simulink model "RC_control"  (Simulink 6.6)
settings: Solver=FixedStepDiscrete  StartTime=0.0  StopTime=10.0  FixedStep=0.001  RelTol=1e-3
undefined symbols (not defined in the file): DiscIntNeverNeededParam, ecan1_init, ecan1_transmit_matlab, OC2max, u1
libraries: simulink x26, dsPICdrivers x11
(part 1 of 2)
settings Model: Creator=Administrator  LastModifiedBy=bwmairs  ProdHWDeviceType=16-bit Generic
settings OptimizationCC: OptimizeModelRefInitCode=on  LifeSpan=1
settings HardwareCC: ProdBitPerInt=16  ProdEndianess=LittleEndian  ProdWordSize=16  ProdHWDeviceType=16-bit Generic  TargetHWDeviceType=32-bit Generic
settings RTWCC: SystemTargetFile=dspic.tlc  TemplateMakefile=dspic_pic30_gcc.tmf  PostCodeGenCommand=dsPIC_Compile()  Description=Embedded Target for Microchip dsPIC (real-time)  ProcessScript=dspic_make_rtw_hook
settings RTWCC: CustomSource=|
  | ../../../../ecan/circBuffer.c
  | ../../../../ecan/ecanFunctions.c
settings RTWCC: CustomInitializer=|
  | #include "InCap.h"
  | #include <p33fxxxx.h>
  |     T5CONbits.TON = 0; // Stop any 16-bit Timer5 operation
  |     T4CONbits.TON = 0; // Stop any 16/32-bit Timer4 operation
  |     T4CONbits.T32 = 1; // Enable 32-bit Timer mode
  |     T4CONbits.TCS = 0; // Select internal instruction cycle clock
  |     T4CONbits.TGATE = 0; // Disable Gated Timer mode
  |     T4CONbits.TCKPS = 0b00;// Select 1:1 Prescaler
  |     TMR5 = 0x00; // Clear 32-bit Timer (msw)
  |     TMR4 = 0x00; // Clear 32-bit Timer (lsw)
  |     PR5 = 0x0010; // Load 32-bit period value (msw)
  |     PR4 = 0x0000; // Load 32-bit period value (lsw)
  |     IPC7bits.T5IP = 0x01; // Set Timer5 Interrupt Priority Level
  |     IFS1bits.T5IF = 0; // Clear Timer5 Interrupt Flag
  |     IEC1bits.T5IE = 1; // Enable Timer5 interrupt
  |     T4CONbits.TON = 1; // Start 32-bit Timer
  | 
  |     // Configure our input captures
  |     OpenCapture1(IC_IDLE_CON & IC_TIMER2_SRC & IC_INT_1CAPTURE &
  |                  IC_EVERY_RISE_EDGE);
  |     ConfigIntCapture1(IC_INT_ON & IC_INT_PRIOR_7);
  |     OpenCapture2(IC_IDLE_CON & IC_TIMER2_SRC & IC_INT_1CAPTURE &
  |                  IC_EVERY_RISE_EDGE);
  |     ConfigIntCapture2(IC_INT_ON & IC_INT_PRIOR_7);
  | 
  | // Configure ports D1, D5, G9 to be open-drain, as 5V outputs are needed
  | ODCGbits.ODCG9 = 1;
  | ODCDbits.ODCD5 = 1;
  | ODCDbits.ODCD1 = 1;
  | 
  | // Enable serial output
  | U2STAbits.UTXEN = 1;
settings CodeAppCC: IgnoreCustomStorageClasses=off
settings STFCustomTargetCC: TargetFcnLib=ansi_tfl_tmw.mat  GenFloatMathFcnCalls=ANSI_C  ModelReferenceCompliant=off  IncludeMdlTerminateFcn=off  CombineOutputUpdateFcns=on  SuppressErrorStatus=on  ERTCustomFileBanners=on  SupportContinuousTime=off  SupportNonInlinedSFcns=off  SystemTargetFile=dspic.tlc
settings ERTTargetCC: TargetFcnLib=ansi_tfl_tmw.mat  GenFloatMathFcnCalls=ANSI_C  ModelReferenceCompliant=off  IncludeMdlTerminateFcn=off  SuppressErrorStatus=on  ModelStepFunctionPrototypeControlCompliant=off  ExtModeMexFile=noextcomm  InlinedParameterPlacement=NonHierarchical  ERTSrcFileBannerTemplate=dsPIC_code_template.cgt  ERTHdrFileBannerTemplate=dsPIC_code_template.cgt  ERTDataSrcFileTemplate=dsPIC_code_template.cgt  ERTDataHdrFileTemplate=dsPIC_code_template.cgt  ERTCustomFileTemplate=dsPIC_main.tlc
settings CustomProperty: DataType=string  Value=C:\PROGRA~1\MATLAB\R2007a\bin\win32\gmake

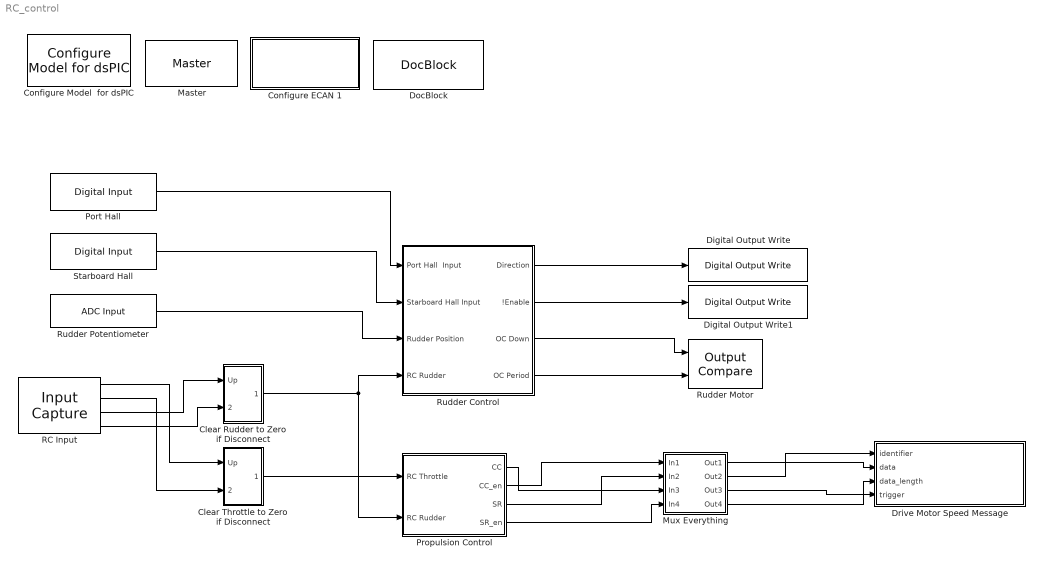
== system RC_control ==
  Clear Rudder to Zero if Disconnect : Subsystem
  Clear Throttle to Zero if Disconnect : Subsystem
  Configure ECAN 1 : Subsystem  mask(Initialize ECAN 1){frame_setting=off, mode=Normal, dma_rx_chan=2, dma_tx_chan=0, baud=250000, ps1=8, pd=5, ps2=6, sjw=4, tq=20, triple_sample=on, dma_buf_size=6 buffers, rx_bufs=[], tx_bufs=[0], buf_0_tx_pri=Highest, buf_0_rte=No, buf_1_tx_pri=Highest, buf_1_rte=No, buf_2_tx_pri=Lowest, buf_2_rte=No, buf_3_tx_pri=Lowest, buf_3_rte=No, buf_4_tx_pri=Lowest, buf_4_rte=No, buf_5_tx_pri=Lowest, buf_5_rte=No, buf_6_tx_pri=Lowest, buf_6_rte=No, buf_7_tx_pri=Lowest, buf_7_rte=No, mask_0=0, mask_0_mide=Match std or ext, mask_1=0, mask_1_mide=Match std or ext, mask_2=0, mask_2_mide=Match std or ext, filters=[], filter_0=hex2dec('400'), filter_0_mask=0, filter_0_exide=Match only standard, filter_0_buf=1, filter_1=hex2dec('401'), filter_1_mask=0, filter_1_exide=Match only standard, filter_1_buf=2, filter_2=hex2dec('402'), filter_2_mask=0, filter_2_exide=Match only standard, filter_2_buf=3, filter_3=0, filter_3_mask=0, filter_3_exide=Match only standard, filter_3_buf=0, filter_4=0, filter_4_mask=0, filter_4_exide=Match only standard, filter_4_buf=0, filter_5=0, filter_5_mask=0, filter_5_exide=Match only standard, filter_5_buf=0, filter_6=0, filter_6_mask=0, filter_6_exide=Match only standard, filter_6_buf=0, filter_7=0, filter_7_mask=0, filter_7_exide=Match only standard, filter_7_buf=0, filter_8=0, filter_8_mask=0, filter_8_exide=Match only standard, filter_8_buf=0, filter_9=0, filter_9_mask=<empty>, filter_9_exide=Match only standard, filter_9_buf=0, filter_10=0, filter_10_mask=0, filter_10_exide=Match only standard, filter_10_buf=0, filter_11=0, filter_11_mask=0, filter_11_exide=Match only standard, filter_11_buf=0, filter_12=0, filter_12_mask=0, filter_12_exide=Match only standard, filter_12_buf=0, filter_13=0, filter_13_mask=0, filter_13_exide=Match only standard, filter_13_buf=0, filter_14=0, filter_14_mask=0, filter_14_exide=Match only standard, filter_14_buf=0, filter_15=0, filter_15_mask=0, filter_15_exide=Match only standard, filter_15_buf=0}
      mask prompts: frame_setting "Extended Frames (Standard if unchecked)"; dma_rx_chan "DMA Reception Channel"; dma_tx_chan "DMA Transmission Channel"; baud "Baud Rate (bps)"; ps1 "Phase Segment 1"; pd "Propagation Delay"; ps2 "Phase Segment 2"; sjw "Sync Jump Width"; tq "Time Quanta"; triple_sample "Triple-sample"; dma_buf_size "DMA Buffer Size"; rx_bufs "Reception Buffers"; tx_bufs "Transmission Buffers"; buf_0_tx_pri "Buffer 0 Transmission Priority"; buf_0_rte "Buffer 0 Remote Transmit Enable"; buf_1_tx_pri "Buffer 1 Transmission Priority"; buf_1_rte "Buffer 1 Remote Transmit Enable"; buf_2_tx_pri "Buffer 2 Transmission Priority"; buf_2_rte "Buffer 2 Remote Transmit Enable"; buf_3_tx_pri "Buffer 3 Transmission Priority"; buf_3_rte "Buffer 3 Remote Transmit Enable"; buf_4_tx_pri "Buffer 4 Transmission Priority"; buf_4_rte "Buffer 4 Remote Transmit Enable"; buf_5_tx_pri "Buffer 5 Transmission Priority"; buf_5_rte "Buffer 5 Remote Transmit Enable"; buf_6_tx_pri "Buffer 6 Transmission Priority"; buf_6_rte "Buffer 6 Remote Transmit Enable"; buf_7_tx_pri "Buffer 7 Transmission Priority"; buf_7_rte "Buffer 7 Remote Transmit Enable"; mask_0 "Mask 0"; mask_0_mide "Mask 0 Receive Mode"; mask_1 "Mask 1"; mask_1_mide "Mask 1 Receive Mode"; mask_2 "Mask 2"; mask_2_mide "Mask 2 Receive Mode"; filter_0 "Filter 0"; filter_0_mask "Filter 0 Mask"; filter_0_exide "Filter 0 Mode"; filter_0_buf "Filter 0 Buffer"; filter_1 "Filter 1"; filter_1_mask "Filter 1 Mask"; filter_1_exide "Filter 1 Mode"; filter_1_buf "Filter 1 Buffer"; filter_2 "Filter 2"; filter_2_mask "Filter 2 Mask"; filter_2_exide "Filter 2 Mode"; filter_2_buf "Filter 2 Buffer"; filter_3 "Filter 3"; filter_3_mask "Filter 3 Mask"; filter_3_exide "Filter 3 Mode"; filter_3_buf "Filter 3 Buffer"; filter_4 "Filter 4"; filter_4_mask "Filter 4 Mask"; filter_4_exide "Filter 4 Mode"; filter_4_buf "Filter 4 Buffer"; filter_5 "Filter 5"; filter_5_mask "Filter 5 Mask"; filter_5_exide "Filter 5 Mode"; filter_5_buf "Filter 5 Buffer"; filter_6 "Filter 6"; filter_6_mask "Filter 6 Mask"; filter_6_exide "Filter 6 Mode"; filter_6_buf "Filter 6 Buffer"; filter_7 "Filter 7"; filter_7_mask "Filter 7 Mask"; filter_7_exide "Filter 7 Mode"; filter_7_buf "Filter 7 Buffer"; filter_8 "Filter 8"; filter_8_mask "Filter 8 Mask"; filter_8_exide "Filter 8 Mode"; filter_8_buf "Filter 8 Buffer"; filter_9 "Filter 9"; filter_9_mask "Filter 9 Mask"; filter_9_exide "Filter 9 Mode"; filter_9_buf "Filter 9 Buffer"; filter_10 "Filter 10"; filter_10_mask "Filter 10 Mask"; filter_10_exide "Filter 10 Mode"; filter_10_buf "Filter 10 Buffer"; filter_11 "Filter 11"; filter_11_mask "Filter 11 Mask"; filter_11_exide "Filter 11 Mode"; filter_11_buf "Filter 11 Buffer"; filter_12 "Filter 12"; filter_12_mask "Filter 12 Mask"; filter_12_exide "Filter 12 Mode"; filter_12_buf "Filter 12 Buffer"; filter_13 "Filter 13"; filter_13_mask "Filter 13 Mask"; filter_13_exide "Filter 13 Mode"; filter_13_buf "Filter 13 Buffer"; filter_14 "Filter 14"; filter_14_mask "Filter 14 Mask"; filter_14_exide "Filter 14 Mode"; filter_14_buf "Filter 14 Buffer"; filter_15 "Filter 15"; filter_15_mask "Filter 15 Mask"; filter_15_exide "Filter 15 Mode"; filter_15_buf "Filter 15 Buffer"
      mask help: Initializes the ECAN 1 module on the dsPIC33f. Allows for configuration of almost all ECAN options to produce a usable system.
      mask init:
      | parameters = uint16(zeros(53,1));
      | 
      | %% Generate parameter 1
      | parameters(1) = frame_setting;
      | mode_id = 0;
      | switch mode
      |     case 'Disabled'
      |         mode_id = 1;
      |     case 'Loopback'
      |         mode_id = 2;
      |     case 'Listen only'
      |         mode_id = 3;
      |     case 'Listen all'
      |         mode_id = 7;
      | end
      | parameters(1) = bitor(parameters(1), bitshift(mode_id, 2));
      | parameters(1) = bitor(parameters(1), bitshift(dma_rx_chan, 5));
      | parameters(1) = bitor(parameters(1), bitshift(dma_tx_chan, 8));
      | 
      | %% Generate parameter 2
      | parameters(2) = baud / 100;
      | 
      | %% Generate parameter 3
      | h = find_system(bdroot(gcb),'FollowLinks','on','LookUnderMasks','all','Tag','dsPIC_MASTER');
      | fcy = 0;
      | if ~isempty(h)
      |     OverrideFcy = strcmp(get_param(h{1},'OverrideFcy'),'on');
      |     if (OverrideFcy == 1)
      |         fcy = str2num(get_param(h{1},'NewFcy'));     %% overridded fcy
      |     else
      |         fcy = str2num(get_param(h{1},'fcy'));
      |     end 
      | end
      | parameters(3) = fcy / 1000;
      | 
      | %% Generate parameter 4
      | parameters(4) = ps1 - 1;
      | parameters(4) = bitor(parameters(4), bitshift(pd - 1, 3));
      | parameters(4) = bitor(parameters(4), bitshift(ps2 - 1, 6));
      | parameters(4) = bitor(parameters(4), bitshift(sjw - 1, 9));
      | if triple_sample == 1
      |     parameters(4) = bitset(parameters(4),12);
      | end
      | 
      | %% Generate parameter 5
      | for k = 1:length(filters)
      |     parameters(5) = bitset(parameters(5),filters(k)+1);
      | end;
      | 
      | % Map filter mask values into proper values
      | filter_masks = [filter_0_mask; filter_1_mask; filter_2_mask; filter_3_mask; filter_4_mask; filter_5_mask; filter_6_mask; filter_7_mask; filter_8_mask; filter_9_mask; filter_10_mask; filter_11_mask; filter_12_mask; filter_13_mask; filter_14_mask; filter_15_mask;];
      | filter_masks = filter_masks - 2;
      | filter_masks(filter_masks == -1) = 3;
      | 
      | %% Generate parameters 6 and 7
      | for k = 1:length(filters);
      |     filter = filters(k) + 1;
      |     if filter < 9
      |         parameters(6) = bitor(parameters(6), bitshift(filter_masks(filter),2*(filter-1)));
      |     else
      |         parameters(7) = bitor(parameters(7), bitshift(filter_masks(filter),2*(filter-9)));
      |     end
      | end
      | 
      | % Generate parameters 8 and 9
      | parameters(8) = bitshift(bitand(mask_0,hex2dec('18000000')),-27); % EID17-16
      | parameters(8) = bitor(parameters(8), bitshift(bitand(mask_0,hex2dec('7FF')), 5)); % SID
      | parameters(8) = bitor(parameters(8), bitshift(mask_0_mide - 1, 3)); % MIDE
      | parameters(9) = bitshift(bitand(mask_0,hex2dec('7FFF800')),-11); % EID15-0
      | 
      | %% Generate parameters 10 and 11
      | parameters(10) = bitshift(bitand(mask_1,hex2dec('18000000')),-27); % EID17-16
      | parameters(10) = bitor(parameters(10), bitshift(bitand(mask_1,hex2dec('7FF')), 5)); % SID
      | parameters(10) = bitor(parameters(10), bitshift(mask_1_mide - 1, 3)); % MIDE
      | parameters(11) = bitshift(bitand(mask_1,hex2dec('7FFF800')),-11); % EID15-0
      | 
      | %% Generate parameters 12 and 13
      | parameters(12) = bitshift(bitand(mask_2,hex2dec('18000000')),-27); % EID17-16
      | parameters(12) = bitor(parameters(12), bitshift(bitand(mask_2,hex2dec('7FF')), 5)); % SID
      | parameters(12) = bitor(parameters(12), bitshift(mask_2_mide - 1, 3)); % MIDE
      | parameters(13) = bitshift(bitand(mask_2,hex2dec('7FFF800')),-11); % EID15-0
      | 
      | % Generate parameters 14-17
      | buf_priorities = [buf_0_tx_pri;buf_1_tx_pri;buf_2_tx_pri;buf_3_tx_pri;buf_4_tx_pri;buf_5_tx_pri;buf_6_tx_pri;buf_7_tx_pri] - 1;
      | buf_rtes = [buf_0_rte;buf_1_rte;buf_2_rte;buf_3_rte;buf_4_rte;buf_5_rte;buf_6_rte;buf_7_rte] - 1;
      | 
      | % Create a vector of chars to modify
      | regs = uint16(zeros(8,1));
      | 
      | % Go through all enabled transmission buffers setting appropriate bits
      | for b = 1:size(tx_bufs,1)
      |     
      |     index = tx_bufs(b) + 1;
      |     
      |     % Set transmission bit
      |     regs(index) = bitset(regs(index),8);
      | 
      |     % Set priority bits
      |     regs(index) = bitor(regs(index), buf_priorities(index));
      | 
      |     % Set remote transmit enable bits
      |     if buf_rtes(index) == 1
      |         regs(index) = bitset(regs(index),3);
      |     end
      | end
      | 
      | for b = 1:size(rx_bufs,1)
      |     
      |     index = rx_bufs(b) + 1;
      | 
      |     % Set priority bits
      |     regs(index) = bitor(regs(index), buf_priorities(index));
      | 
      |     % Set remote transmit enable bits
      |     if buf_rtes(index) == 1
      |         regs(index) = bitset(regs(index),3);
      |     end
      | end
      | 
      | % Map our matrix into registers
      | parameters(14) = bitor(bitshift(regs(2),8), regs(1));
      | parameters(15) = bitor(bitshift(regs(4),8), regs(3));
      | parameters(16) = bitor(bitshift(regs(6),8), regs(5));
      | parameters(17) = bitor(bitshift(regs(8),8), regs(7));
      | 
      | % Map the filter buffer values to corresponding bit values
      | filter_buffers = [filter_0_buf; filter_1_buf; filter_2_buf; filter_3_buf; filter_4_buf; filter_5_buf; filter_6_buf; filter_7_buf; filter_8_buf; filter_9_buf; filter_10_buf; filter_11_buf; filter_12_buf; filter_13_buf; filter_14_buf; filter_15_buf;];
      | filter_buffers = filter_buffers - 1;
      | 
      | %% Generate parameter 18
      | if bitget(parameters(5),1) == 1
      |     parameters(18) = filter_buffers(1);
      | end
      | if bitget(parameters(5),2) == 1
      |     parameters(18) = bitor(parameters(18), bitshift(filter_buffers(2), 4));
      | end
      | if bitget(parameters(5),3) == 1
      |     parameters(18) = bitor(parameters(18), bitshift(filter_buffers(3), 8));
      | end
      | if bitget(parameters(5),4) == 1
      |     parameters(18) = bitor(parameters(18), bitshift(filter_buffers(4), 12));
      | end
      | 
      | %% Generate parameter 19
      | if bitget(parameters(5),5) == 1
      |     parameters(19) = filter_buffers(5);
      | end
      | if bitget(parameters(5),6) == 1
      |     parameters(19) = bitor(parameters(19), bitshift(filter_buffers(6), 4));
      | end
      | if bitget(parameters(5),7) == 1
      |     parameters(19) = bitor(parameters(19), bitshift(filter_buffers(7), 8));
      | end
      | if bitget(parameters(5),8) == 1
      |     parameters(19) = bitor(parameters(19), bitshift(filter_buffers(8), 12));
      | end
      | 
      | %% Generate parameter 20
      | if bitget(parameters(5),9) == 1
      |     parameters(20) = filter_buffers(9);
      | end
      | if bitget(parameters(5),10) == 1
      |     parameters(20) = bitor(parameters(20), bitshift(filter_buffers(10), 4));
      | end
      | if bitget(parameters(5),11) == 1
      |     parameters(20) = bitor(parameters(20), bitshift(filter_buffers(11), 8));
      | end
      | if bitget(parameters(5),12) == 1
      |     parameters(20) = bitor(parameters(20), bitshift(filter_buffers(12), 12));
      | end
      | 
      | %% Generate parameter 21
      | if bitget(parameters(5),13) == 1
      |     parameters(21) = filter_buffers(13);
      | end
      | if bitget(parameters(5),14) == 1
      |     parameters(21) = bitor(parameters(21), bitshift(filter_buffers(14), 4));
      | end
      | if bitget(parameters(5),15) == 1
      |     parameters(21) = bitor(parameters(21), bitshift(filter_buffers(15), 8));
      | end
      | if bitget(parameters(5),16) == 1
      |     parameters(21) = bitor(parameters(21), bitshift(filter_buffers(16), 12));
      | end
      | 
      | % Generate parameters 22 and 23
      | parameters(22) = bitshift(bitand(filter_0,hex2dec('18000000')),-27); % EID17-16
      | parameters(22) = bitor(parameters(22), bitshift(bitand(filter_0,hex2dec('7FF')), 5)); % SID
      | parameters(22) = bitor(parameters(22), bitshift(filter_0_exide - 1, 3)); % EXIDE
      | parameters(23) = bitshift(bitand(uint32(filter_0),hex2dec('7FFF800')),-11); % EID15-0
      | 
      | %% Generate parameters 24 and 25
      | parameters(24) = bitshift(bitand(filter_1,hex2dec('18000000')),-27); % EID17-16
      | parameters(24) = bitor(parameters(24), bitshift(bitand(filter_1,hex2dec('7FF')), 5)); % SID
      | parameters(24) = bitor(parameters(24), bitshift(filter_1_exide - 1, 3)); % EXIDE
      | parameters(25) = bitshift(bitand(uint32(filter_1),hex2dec('7FFF800')),-11); % EID15-0
      | 
      | %% Generate parameters 26 and 27
      | parameters(26) = bitshift(bitand(filter_2,hex2dec('18000000')),-27); % EID17-16
      | parameters(26) = bitor(parameters(26), bitshift(bitand(filter_2,hex2dec('7FF')), 5)); % SID
      | parameters(26) = bitor(parameters(26), bitshift(filter_2_exide - 1, 3)); % EXIDE
      | parameters(27) = bitshift(bitand(uint32(filter_2),hex2dec('7FFF800')),-11); % EID15-0
      | 
      | %% Generate parameters 28 and 29
      | parameters(28) = bitshift(bitand(filter_3,hex2dec('18000000')),-27); % EID17-16
      | parameters(28) = bitor(parameters(28), bitshift(bitand(filter_3,hex2dec('7FF')), 5)); % SID
      | parameters(28) = bitor(parameters(28), bitshift(filter_3_exide - 1, 3)); % EXIDE
      | parameters(29) = bitshift(bitand(uint32(filter_3),hex2dec('7FFF800')),-11); % EID15-0
      | 
      | %% Generate parameters 30 and 31
      | parameters(30) = bitshift(bitand(filter_4,hex2dec('18000000')),-27); % EID17-16
      | parameters(30) = bitor(parameters(30), bitshift(bitand(filter_4,hex2dec('7FF')), 5)); % SID
      | parameters(30) = bitor(parameters(30), bitshift(filter_4_exide - 1, 3)); % EXIDE
      | parameters(31) = bitshift(bitand(uint32(filter_4),hex2dec('7FFF800')),-11); % EID15-0
      | 
      | %% Generate parameters 32 and 33
      | parameters(32) = bitshift(bitand(filter_5,hex2dec('18000000')),-27); % EID17-16
      | parameters(32) = bitor(parameters(32), bitshift(bitand(filter_5,hex2dec('7FF')), 5)); % SID
      | parameters(32) = bitor(parameters(32), bitshift(filter_5_exide - 1, 3)); % EXIDE
      | parameters(33) = bitshift(bitand(uint32(filter_5),hex2dec('7FFF800')),-11); % EID15-0
      | 
      | %% Generate parameters 34 and 35
      | parameters(34) = bitshift(bitand(filter_6,hex2dec('18000000')),-27); % EID17-16
      | parameters(34) = bitor(parameters(34), bitshift(bitand(filter_6,hex2dec('7FF')), 5)); % SID
      | parameters(34) = bitor(parameters(34), bitshift(filter_6_exide - 1, 3)); % EXIDE
      | parameters(35) = bitshift(bitand(uint32(filter_6),hex2dec('7FFF800')),-11); % EID15-0
      | 
      | %% Generate parameters 36 and 37
      | parameters(36) = bitshift(bitand(filter_7,hex2dec('18000000')),-27); % EID17-16
      | parameters(36) = bitor(parameters(36), bitshift(bitand(filter_7,hex2dec('7FF')), 5)); % SID
      | parameters(36) = bitor(parameters(36), bitshift(filter_7_exide - 1, 3)); % EXIDE
      | parameters(37) = bitshift(bitand(uint32(filter_7),hex2dec('7FFF800')),-11); % EID15-0
      | 
      | %% Generate parameters 38 and 39
      | parameters(38) = bitshift(bitand(filter_8,hex2dec('18000000')),-27); % EID17-16
      | parameters(38) = bitor(parameters(38), bitshift(bitand(filter_8,hex2dec('7FF')), 5)); % SID
      | parameters(38) = bitor(parameters(38), bitshift(filter_8_exide - 1, 3)); % EXIDE
      | parameters(39) = bitshift(bitand(uint32(filter_8),hex2dec('7FFF800')),-11); % EID15-0
      | 
      | %% Generate parameters 40 and 41
      | parameters(40) = bitshift(bitand(filter_9,hex2dec('18000000')),-27); % EID17-16
      | parameters(40) = bitor(parameters(40), bitshift(bitand(filter_9,hex2dec('7FF')), 5)); % SID
      | parameters(40) = bitor(parameters(40), bitshift(filter_9_exide - 1, 3)); % EXIDE
      | parameters(41) = bitshift(bitand(uint32(filter_9),hex2dec('7FFF800')),-11); % EID15-0
      | 
      | %% Generate parameters 42 and 43
      | parameters(42) = bitshift(bitand(filter_10,hex2dec('18000000')),-27); % EID17-16
      | parameters(42) = bitor(parameters(42), bitshift(bitand(filter_10,hex2dec('7FF')), 5)); % SID
      | parameters(42) = bitor(parameters(42), bitshift(filter_10_exide - 1, 3)); % EXIDE
      | parameters(43) = bitshift(bitand(uint32(filter_10),hex2dec('7FFF800')),-11); % EID15-0
      | 
      | %% Generate parameters 44 and 45
      | parameters(44) = bitshift(bitand(filter_11,hex2dec('18000000')),-27); % EID17-16
      | parameters(44) = bitor(parameters(44), bitshift(bitand(filter_11,hex2dec('7FF')), 5)); % SID
      | parameters(44) = bitor(parameters(44), bitshift(filter_11_exide - 1, 3)); % EXIDE
      | parameters(45) = bitshift(bitand(uint32(filter_11),hex2dec('7FFF800')),-11); % EID15-0
      | 
      | %% Generate parameters 46 and 47
      | parameters(46) = bitshift(bitand(filter_12,hex2dec('18000000')),-27); % EID17-16
      | parameters(46) = bitor(parameters(46), bitshift(bitand(filter_12,hex2dec('7FF')), 5)); % SID
      | parameters(46) = bitor(parameters(46), bitshift(filter_12_exide - 1, 3)); % EXIDE
      | parameters(47) = bitshift(bitand(uint32(filter_12),hex2dec('7FFF800')),-11); % EID15-0
      | 
      | %% Generate parameters 48 and 49
      | parameters(48) = bitshift(bitand(filter_13,hex2dec('18000000')),-27); % EID17-16
      | parameters(48) = bitor(parameters(48), bitshift(bitand(filter_13,hex2dec('7FF')), 5)); % SID
      | parameters(48) = bitor(parameters(48), bitshift(filter_13_exide - 1, 3)); % EXIDE
      | parameters(49) = bitshift(bitand(uint32(filter_13),hex2dec('7FFF800')),-11); % EID15-0
      | 
      | %% Generate parameters 50 and 51
      | parameters(50) = bitshift(bitand(filter_14,hex2dec('18000000')),-27); % EID17-16
      | parameters(50) = bitor(parameters(50), bitshift(bitand(filter_14,hex2dec('7FF')), 5)); % SID
      | parameters(50) = bitor(parameters(50), bitshift(filter_14_exide - 1, 3)); % EXIDE
      | parameters(51) = bitshift(bitand(uint32(filter_14),hex2dec('7FFF800')),-11); % EID15-0
      | 
      | %% Generate parameters 52 and 53
      | parameters(52) = bitshift(bitand(filter_15,hex2dec('18000000')),-27); % EID17-16
      | parameters(52) = bitor(parameters(52), bitshift(bitand(filter_15,hex2dec('7FF')), 5)); % SID
      | parameters(52) = bitor(parameters(52), bitshift(filter_15_exide - 1, 3)); % EXIDE
      | parameters(53) = bitshift(bitand(uint32(filter_15),hex2dec('7FFF800')),-11); % EID15-0
      mask StyleString: checkbox,popup(Disabled|Listen all|Listen only|Loopback|Normal),edit,edit,edit,edit,edit,edit,popup(1|2|3|4),edit,checkbox,popup(4 buffers|6 buffers|8 buffers|12 buffers|16 buffers|24 buffers|32 buffers),edit,edit,popup(Lowest|Low|High|Highest),popup(No|Yes),popup(Lowest|Low|High|Highest),popup(No|Yes),popup(Lowest|Low|High|Highest),popup(No|Yes),popup(Lowest|Low|High|Highest),popup(No|Yes),popup(Lowest|Low|High|Highest),popup(No|Yes),popup(Lowest|Low|High|Highest),popup(No|Yes),popup(Lowest|Low|High|Highest),popup(No|Yes),popup(Lowest|Low|High|Highest),popup(No|Yes),edit,popup(Match std or ext|Obey filter mode),edit,popup(Match std or ext|Obey filter mode),edit,popup(Match std or ext|Obey filter mode),edit,edit,popup(--|0|1|2),popup(Match only standard|Match only extended),popup(0|1|2|3|4|5|6|7|8|9|10|11|12|13|14|FIFO),edit,popup(--|0|1|2),popup(Match only standard|Match only extended),popup(0|1|2|3|4|5|6|7|8|9|10|11|12|13|14|FIFO),edit,popup(--|0|1|2),popup(Match only standard|Match only extended),popup(0|1|2|3|4|5|6|7|8|9|10|11|12|13|14|FIFO),edit,popup(--|0|1|2),popup(Match only standard|Match only extended),popup(0|1|2|3|4|5|6|7|8|9|10|11|12|13|14|FIFO),edit,popup(--|0|1|2),popup(Match only standard|Match only extended),popup(0|1|2|3|4|5|6|7|8|9|10|11|12|13|14|FIFO),edit,popup(--|0|1|2),popup(Match only standard|Match only extended),popup(0|1|2|3|4|5|6|7|8|9|10|11|12|13|14|FIFO),edit,popup(--|0|1|2),popup(Match only standard|Match only extended),popup(0|1|2|3|4|5|6|7|8|9|10|11|12|13|14|FIFO),edit,popup(--|0|1|2),popup(Match only standard|Match only extended),popup(0|1|2|3|4|5|6|7|8|9|10|11|12|13|14|FIFO),edit,popup(--|0|1|2),popup(Match only standard|Match only extended),popup(0|1|2|3|4|5|6|7|8|9|10|11|12|13|14|FIFO),edit,popup(<empty>),popup(Match only standard|Match only extended),popup(0|1|2|3|4|5|6|7|8|9|10|11|12|13|14|FIFO),edit,popup(--|0|1|2),popup(Match only standard|Match only extended),popup(0|1|2|3|4|5|6|7|8|9|10|11|12|13|14|FIFO),edit,popup(--|0|1|2),popup(Match only standard|Match only extended),popup(0|1|2|3|4|5|6|7|8|9|10|11|12|13|14|FIFO),edit,popup(--|0|1|2),popup(Match only standard|Match only extended),popup(0|1|2|3|4|5|6|7|8|9|10|11|12|13|14|FIFO),edit,popup(--|0|1|2),popup(Match only standard|Match only extended),popup(0|1|2|3|4|5|6|7|8|9|10|11|12|13|14|FIFO),edit,popup(--|0|1|2),popup(Match only standard|Match only extended),popup(0|1|2|3|4|5|6|7|8|9|10|11|12|13|14|FIFO),edit,popup(--|0|1|2),popup(Match only standard|Match only extended),popup(0|1|2|3|4|5|6|7|8|9|10|11|12|13|14|FIFO)
      mask CallbackString:
      | |||||tq = 1 + str2num(get_param(gcb, 'ps1')) + str2num(get_param(gcb, 'pd')) + str2num(get_param(gcb, 'ps2'));
      | set_param(gcb, 'tq', int2str(tq));|tq = 1 + str2num(get_param(gcb, 'ps1')) + str2num(get_param(gcb, 'pd')) + str2num(get_param(gcb, 'ps2'));
      | set_param(gcb, 'tq', int2str(tq));|tq = 1 + str2num(get_param(gcb, 'ps1')) + str2num(get_param(gcb, 'pd')) + str2num(get_param(gcb, 'ps2'));
      | set_param(gcb, 'tq', int2str(tq));||||||filters = eval(get_param(gcb,'tx_bufs'));
      | mVisibilities = get_param(gcb,'MaskVisibilities');
      | mNames = get_param(gcb,'MaskNames');
      | for i = 1:size(mNames);
      | 	n = mNames{i};
      |     if size(n,2) > 4 && strcmp(n(1:4), 'buf_') == 1
      |         filterNumber = sscanf(n, 'buf_%d');
      |         if isempty(find(filters == filterNumber, 1)) == 0
      |              mVisibilities{i} = 'on';
      |         else
      |              mVisibilities{i} = 'off';
      |         end
      |     end
      | end
      | set_param(gcb, 'MaskVisibilities', mVisibilities);|||||||||||||||||||||||filters = eval(get_param(gcb,'filters'));
      | mVisibilities = get_param(gcb,'MaskVisibilities');
      | mNames = get_param(gcb,'MaskNames');
      | for i = 1:size(mNames);
      | 	n = mNames{i};
      |     if size(n,2) > 7 && strcmp(n(1:7), 'filter_') == 1
      |         filterNumber = sscanf(n, 'filter_%d');
      |         if isempty(find(filters == filterNumber, 1)) == 0
      |              mVisibilities{i} = 'on';
      |         else
      |              mVisibilities{i} = 'off';
      |         end
      |     end
      | end
      | set_param(gcb, 'MaskVisibilities', mVisibilities);||||||||||||||||||||||||||||||||||||||||||||||||||||||||||||||||
      mask Display: text(0.5,0.5,'Configure ECAN1','horizontalAlignment','center','verticalAlignment','middle');
  Configure Model  for dsPIC : dsPICdrivers/Simulink Configuration/Configure Model  for dsPIC
  Digital Output Write : dsPICdrivers/Digital I//O/Digital Output Write  Tag=dsPIC_Digital_Output  Priority=5  PORT=D  Pin=[5]  Simultaneous=off  OrderingInOutPopup=None
  Digital Output Write1 : dsPICdrivers/Digital I//O/Digital Output Write  Tag=dsPIC_Digital_Output  Priority=5  PORT=G  Pin=[9]  Simultaneous=off  OrderingInOutPopup=None
  DocBlock : simulink/Model-Wide Utilities/DocBlock  SystemSampleTime=-1  DocumentType=Text
      content=|
      | This system is designed for use with the Explorer 16 board. It requires the following connections:
      | Port D8 - (input) PWM input for throttle from RC receiver (2ms high = max forward, 1ms high = max reverse)
      | Port D9 - (input) PWM input for rudder from RC receiver (2ms high = hard port, 1ms high = hard stern)
      | Port F3 - (input) Port Hall Effect Sensor
      | Port B0 - (input) Position pot for the rudder
      | Port G3 - (input) Starboard Hall Effect Sensor
      | Port OC2/RD1 - (output) Step output for rudder driver board
      | Port G9 - (output) Enable output for rudder driver board, wired low.
      | Port D5 - (output) Direction output for rudder driver board (Rudder is configured so that a low signal turns to port)
      | Port G0/1 - (output) TX/RX lines for the ECAN peripheral to use CAN1 on the ECAN/LIN PICtail board.
      | Power - connected
      |
      | This model provides remote control for the roboat via standard RC hardware relying on PWM signals.
      | It expects a range of 1.12-2.11V for the rudder position potentiometer with 2.11V being hard to port.
      | This means that the rudder potentiometer should be powered at 3.3V.
      |
      | A failsafe has been implemented, though rather crudely, to detect a loss of RC connection and to
      | reduce propeller speed to zero and disable rudder control. This works by using a 50ms timer that is
      | set every input capture event. If it expires (the 5-channel PWM input we're using have 20ms periods)
      | then we assume there is a loss in connection. Reconnection automatically starts the PWM signals up
      | again and they continue to be read by the dsPIC. The code I am using doesn't seem to work for the
      | first input capture and I'm not certain why at this time. As the clearing event works for both input
      | captures, I am using input capture two to detect a disconnect.
  Drive Motor Speed Message : Subsystem  mask(Send ECAN Message){buffer=0, identifier=hex2dec('301'), identifier_from_input=on, ide=off, remote=off, data=[hex2dec('11') hex2dec('12') hex2dec('13') hex2dec('14')], data_length=4, data_from_input=on, c_func_sample_time=.01, trigger_on_input=on}
      mask prompts: identifier_from_input "Identifier from input"; data_length "Data length"; data_from_input "Data from input"; c_func_sample_time "Sample time"; trigger_on_input "Trigger on input"
      mask help: This block allows for the transmission of a message over the ECAN module.
      mask CallbackString:
      | ||mEnables = get_param(gcb,'MaskEnables');
      | enabled = get_param(gcb, 'identifier_from_input');
      | if strcmp(enabled,'on');
      |     replace_block([gcb '/identifier'],'Constant','Inport','noprompt');
      |     mEnables{2} = 'off';
      |     set_param([gcb '/identifier'],'Port','1');
      | else
      |     replace_block([gcb '/identifier'],'Inport','Constant','noprompt');
      |     mEnables{2} = 'on';
      |     set_param([gcb '/identifier'],'Value','identifier');
      | end
      | set_param(gcb, 'MaskEnables', mEnables);
      | |||data = eval(get_param(gcb, 'data'));
      | y = size(data,1);
      | x = size(data,2);
      | if y > 1 && x > 1
      |     error('Data must be a 1-dimensional vector')
      | else
      |     if or(x > 8, y > 8)
      |         error('Data cannot be larger than 8-bytes');
      |     end
      | end
      | 
      | set_param(gcb, 'data_length', num2str(length(data)));|data_length = eval(get_param(gcb, 'data_length'));
      | if or(data_length < 0, data_length > 9)
      |     error('Data cannot be more than 8 bytes or less than 0.')
      | end|mEnables = get_param(gcb,'MaskEnables');
      | enabled = get_param(gcb, 'data_from_input');
      | if strcmp(enabled,'on');
      |     replace_block([gcb '/data'],'Constant','Inport','noprompt');
      |     replace_block([gcb '/data_length'],'Constant','Inport','noprompt');
      |     mEnables{6} = 'off';
      |     mEnables{7} = 'off';
      |     port = 1;
      |     if ~isempty(find_system(gcb,'LookUnderMasks','all','Name','identifier'))
      |         port = 2;
      |     end
      |     set_param([gcb '/data'],'Port',num2str(port));
      |     set_param([gcb '/data_length'],'Port',num2str(port+1));
      | else
      |     replace_block([gcb '/data'],'Inport','Constant','noprompt');
      |     replace_block([gcb '/data_length'],'Inport','Constant','noprompt');
      |     mEnables{6} = 'on';
      |     mEnables{7} = 'on';
      |     set_param([gcb '/data'],'Value','data');
      |     set_param([gcb '/data'],'OutDataTypeMode','uint8');
      |     set_param([gcb '/data_length'],'Value','data_length');
      |     set_param([gcb '/data_length'],'OutDataTypeMode','uint8');
      | end
      | set_param(gcb, 'MaskEnables', mEnables);
      | ||mEnables = get_param(gcb,'MaskEnables');
      | enabled = get_param(gcb, 'trigger_on_input');
      | c_func_blk = find_system(gcb,'LookUnderMasks','all','FunctionName','dsPIC_C_function_Call');
      | if strcmp(enabled,'on');
      |     mEnables{9} = 'off';
      |     %set_param(c_func_blk,'SampleTime','-1');
      |     replace_block([gcb '/trigger'],'Constant','Inport','noprompt');
      | else
      |     mEnables{9} = 'on';
      |     %set_param(c_func_blk,'SampleTime','c_func_sample_time');
      |     replace_block([gcb '/trigger'],'Inport','Constant','noprompt');
      |     %set_param([gcb '/trigger'],'Value','1');
      | end
      | set_param(gcb, 'MaskEnables', mEnables);
      mask Display: disp('ECAN1 TX');
  Master : dsPICdrivers/Master  Tag=dsPIC_MASTER  Priority=1  TimeStepType=Timer1  picType=33fJ256GP710  fcy=40000000  Quartz_33f=8e6  PLLActive_33f=on  fcyDesired_33f=40000000  tmr1="[1  39999  0]"  tmr1Info="Time Step : 0.001  ;   Error : 0%  PR1=39999"  tmr2345="[8  1  0  0  0  0  0  0]"  tmr2345cfg=[-1 -1 -1 -1 -1 -1 -1 -1]  IOautoConf=on  typePort="[ 0   0   0   0   0   0   0   0   0   0   0   0   0   0   0   0   8   0   0   0   0   0   0   0   0   0   0   0   0   0   0   0   0   0   0   0   0   0   0   0   0   0   0   0   0   0   0   0   0   7   0   0   0  10   0   0   6   6   0   0   0   0   0   0   0   0   0   0   0   0   0   0   0   0   0   0   0   0   0   0   0   0   0   9   0   0   0   0   0   0   0   0   0   0   0   0   0   0   0   9   0   0   0   0   0  10   0   0   0   0   0   0 ]"  TRIS="[ 65535  65535  65535  65501  65535  65535  65023 ]"  ADPCFG=0  MasterBusyPort=None  MasterOverloadPort=None  FOSC=Quartz (XT - HS)  ClockSwitchMonitor=Both disabled  TempProtection_33f=TEMP_ON  FPBOR=<empty>  PWRT=disable  MCLR=<empty>  ICD=ICS_NONE  JTAGEN=JTAGEN_OFF  PowerSave=off  OverrideFcy=off  NewFcy=1e6  PR2345="[65535  65535  65535  65535  65535  65535  65535  65535]"
  Mux Everything : Subsystem
  Port Hall : dsPICdrivers/Digital I//O/Digital Input  Tag=dsPIC_Digital_Input  PORT=F  Pin=[3]  SampleTime=.01  OrderingInOutPopup=None
  Propulsion Control : Subsystem
  RC Input : dsPICdrivers/Peripheral I//O/Input Capture  Tag=dsPIC_PWM_IC  Priority=5  IntPriority=7  Channel=[ 1 2 ]  Channel_UP_Down_Periode="[1  1]"  MaxChannel="[0.001       0.001]"  SafeMarge="[10  10]"  MaxName=' IC1max , IC2max '  Precision="[15.4252      15.4252]"  Timer="[3  3]"  ChangeDetected="[2  2]"  ChangeDetectedPortRef=3  SampleTime=.01  Status=OK
  Rudder Potentiometer : dsPICdrivers/Peripheral I//O/ADC Input  Tag=dsPIC_ADC  Priority=5  ADC_TYPE=10 bits  ADC_MODE=Continuous sampling & get last channel value  NbrSampleStep=1  VoltRefpopup="AVdd  -  AVss"  OutFormatBitspopup=ssss sssd dddd dddd : Signed Integer  InterruptPriority=6  ANCHANNELS=[0]  MaxName=ANmax = 1023  Rin=1e2  ADCS=12  SAMC=1  Temperature=25  DMAChannel=0  SampleTime=.01  Status="OK  |  Tsmp=1.625e-007 |  T/Channel=2.113e-006 |  Tall=2.113e-006"  SSRC=auto convert
  Rudder Control : Subsystem
  Rudder Motor : dsPICdrivers/Peripheral I//O/Output Compare  Tag=dsPIC_PWM_out  Priority=5  IntPriority=3  CHANNEL=[2]  Channel_UP_Down_Periode=[5]  MaxChannel=[0.01]  MaxName=' OC2max '  Precision=[15.6096]  Timer=[2]  Status=OK  SafeMarge=[0]  PortLetter=[68]  PortNumber=[1]  MaxValues=[49999]
  Starboard Hall : dsPICdrivers/Digital I//O/Digital Input  Tag=dsPIC_Digital_Input  PORT=G  Pin=[3]  SampleTime=.01  OrderingInOutPopup=None
  wires:
  Rudder Control/3(OC Down) -> Rudder Motor/1
  Starboard Hall/1 -> Rudder Control/2(Starboard Hall Input)
  Port Hall/1 -> Rudder Control/1(Port Hall  Input)
  Rudder Potentiometer/1 -> Rudder Control/3(Rudder Position)
  Rudder Control/1(Direction) -> Digital Output Write/1
  Rudder Control/4(OC Period) -> Rudder Motor/2
  Rudder Control/2(!Enable) -> Digital Output Write1/1
  Mux Everything/4(Out4) -> Drive Motor Speed Message/3(data_length)
  Clear Throttle to Zero if Disconnect/1(Out) -> Propulsion Control/1(RC Throttle)
  Clear Rudder to Zero if Disconnect/1(Out) -> Rudder Control/4(RC Rudder), Propulsion Control/2(RC Rudder)
  Mux Everything/3(Out3) -> Drive Motor Speed Message/4(trigger)
  Propulsion Control/2(CC_en) -> Mux Everything/1(In1)
  Mux Everything/2(Out2) -> Drive Motor Speed Message/1(identifier)
  Propulsion Control/3(SR) -> Mux Everything/2(In2)
  Propulsion Control/1(CC) -> Mux Everything/3(In3)
  RC Input/3 -> Clear Rudder to Zero if Disconnect/1(Up)
  RC Input/4 -> Clear Rudder to Zero if Disconnect/2(Fall)
  RC Input/2 -> Clear Throttle to Zero if Disconnect/2(Fall)
  RC Input/1 -> Clear Throttle to Zero if Disconnect/1(Up)
  Mux Everything/1(Out1) -> Drive Motor Speed Message/2(data)
  Propulsion Control/4(SR_en) -> Mux Everything/4(In4)

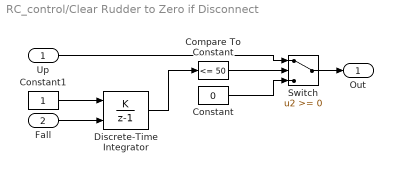
== system RC_control/Clear Rudder to Zero if Disconnect ==
  Up : Inport
  Fall : Inport  Port=2
  Compare To Constant : simulink/Logic and Bit Operations/Compare To Constant  SystemSampleTime=-1  relop=<=  const=50  LogicOutDataTypeMode=boolean  ZeroCross=off
  Constant : Constant  Value=0
  Constant1 : Constant
  Discrete-Time Integrator : DiscreteIntegrator  IntegratorMethod=Accumulation: Forward Euler  ExternalReset=level  SampleTime=-1  ICPrevOutput=DiscIntNeverNeededParam  ICPrevScaledInput=DiscIntNeverNeededParam
  Switch : Switch
  Out : Outport
  wires:
  Constant1/1 -> Discrete-Time Integrator/1
  Compare To Constant/1 -> Switch/2
  Fall/1 -> Discrete-Time Integrator/2
  Switch/1 -> Out/1
  Constant/1 -> Switch/3
  Discrete-Time Integrator/1 -> Compare To Constant/1
  Up/1 -> Switch/1

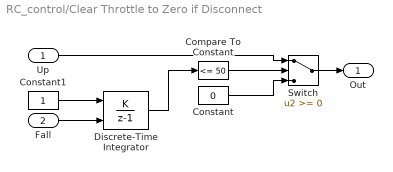
== system RC_control/Clear Throttle to Zero if Disconnect ==
  Up : Inport
  Fall : Inport  Port=2
  Compare To Constant : simulink/Logic and Bit Operations/Compare To Constant  SystemSampleTime=-1  relop=<=  const=50  LogicOutDataTypeMode=boolean  ZeroCross=off
  Constant : Constant  Value=0
  Constant1 : Constant
  Discrete-Time Integrator : DiscreteIntegrator  IntegratorMethod=Accumulation: Forward Euler  ExternalReset=level  SampleTime=-1  ICPrevOutput=DiscIntNeverNeededParam  ICPrevScaledInput=DiscIntNeverNeededParam
  Switch : Switch
  Out : Outport
  wires:
  Up/1 -> Switch/1
  Discrete-Time Integrator/1 -> Compare To Constant/1
  Constant/1 -> Switch/3
  Switch/1 -> Out/1
  Fall/1 -> Discrete-Time Integrator/2
  Compare To Constant/1 -> Switch/2
  Constant1/1 -> Discrete-Time Integrator/1

== system RC_control/Configure ECAN 1 ==
  C Function Call [ecanFunctions.c] : dsPICdrivers/OTHERS/C Function Call  Tag=dsPIC_dsPIC_CFunctionCall  fctName='ecan1_init'  INPUT_SIZE=53  INPUT1=uint16  INPUT2=--  INPUT3=--  OUTPUT_SIZE=1  OUTPUT1=--  SampleTime=Inf  InputType=[ 4 ]  OutputType=[ ]  FctDeclaration=extern void ecan1_init(uint16_T* u1);  FctCall=ecan1_init(*%u1);  OrderingInOutPopup=None
  Constant : Constant  Value=parameters  OutDataTypeMode=uint16
  wires:
  Constant/1 -> C Function Call [ecanFunctions.c]/1

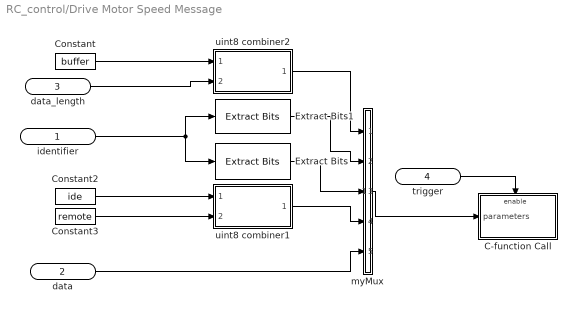
== system RC_control/Drive Motor Speed Message ==
  identifier : Inport
  data : Inport  Port=2
  data_length : Inport  Port=3
  trigger : Inport  Port=4
  C-function Call : Subsystem
  Constant : Constant  Value=buffer  OutDataTypeMode=uint8
  Constant2 : Constant  Value=ide  OutDataTypeMode=uint8
  Constant3 : Constant  Value=remote  OutDataTypeMode=uint8
  Extract Bits : simulink/Logic and Bit Operations/Extract Bits  SystemSampleTime=-1  bitsToExtract=Upper half  numBits=8  bitIdxRange=[0 7]  outScalingMode=Treat bit field as an integer
  Extract Bits1 : simulink/Logic and Bit Operations/Extract Bits  SystemSampleTime=-1  bitsToExtract=Lower half  numBits=8  bitIdxRange=[0 7]  outScalingMode=Preserve fixed-point scaling
  myMux : Stateflow chart
  uint8 combiner1 : Subsystem
  uint8 combiner2 : Subsystem
  wires:
  data/1 -> myMux/5(u5)
  Constant2/1 -> uint8 combiner1/1(high-order)
  Constant3/1 -> uint8 combiner1/2(low-order)
  uint8 combiner1/1(combined) -> myMux/4(u4)
  identifier/1 -> Extract Bits/1, Extract Bits1/1
  Extract Bits1/1 -> myMux/2(u2)
  Extract Bits/1 -> myMux/3(u3)
  data_length/1 -> uint8 combiner2/2(low-order)
  Constant/1 -> uint8 combiner2/1(high-order)
  uint8 combiner2/1(combined) -> myMux/1(u1)
  myMux/1(y) -> C-function Call/1(parameters)
  trigger/1 -> C-function Call/Enable

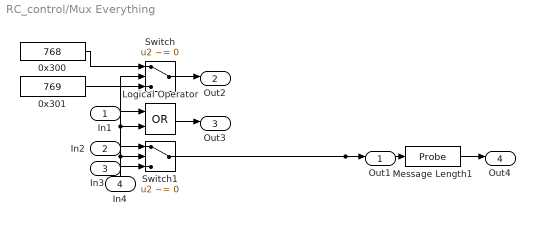
== system RC_control/Mux Everything ==
  In1 : Inport
  In2 : Inport  Port=2
  In3 : Inport  Port=3
  In4 : Inport  Orientation=up  Port=4
  0x300 : Constant  Value=768
  0x301 : Constant  Value=769
  Logical Operator : Logic  Operator=OR  AllPortsSameDT=off  OutDataTypeMode=Boolean
  Message Length1 : Probe  ProbeSampleTime=off  ProbeComplexSignal=off  ProbeWidthDataType=uint8
  Switch : Switch  Criteria=u2 ~= 0
  Switch1 : Switch  Criteria=u2 ~= 0
  Out1 : Outport
  Out2 : Outport  Port=2
  Out3 : Outport  Port=3
  Out4 : Outport  Port=4
  wires:
  In4/1 -> Switch1/2, Switch/2, Logical Operator/2
  0x300/1 -> Switch/1
  0x301/1 -> Switch/3
  Switch1/1 -> Message Length1/1, Out1/1
  Switch/1 -> Out2/1
  In1/1 -> Logical Operator/1
  Logical Operator/1 -> Out3/1
  In2/1 -> Switch1/1
  Message Length1/1 -> Out4/1
  In3/1 -> Switch1/3

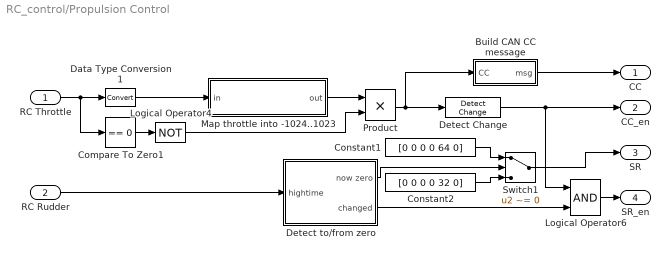
== system RC_control/Propulsion Control ==
  RC Throttle : Inport
  RC Rudder : Inport  Port=2
  Build CAN CC message : Subsystem
  Compare To Zero1 : simulink/Logic and Bit Operations/Compare To Zero  SystemSampleTime=-1  relop===  LogicOutDataTypeMode=boolean  ZeroCross=off
  Constant1 : Constant  Value=[0 0 0 0 64 0]
  Constant2 : Constant  Value=[0 0 0 0 32 0]
  Data Type Conversion1 : DataTypeConversion  OutDataTypeMode=int16
  Detect Change : simulink/Logic and Bit Operations/Detect Change  SystemSampleTime=-1  vinit=0
  Detect to/from zero : Subsystem
  Logical Operator4 : Logic  Operator=NOT  AllPortsSameDT=off  OutDataTypeMode=Boolean
  Logical Operator6 : Logic  AllPortsSameDT=off  OutDataTypeMode=Specify via dialog
  Map throttle into -1024..1023 : Subsystem
  Product : Product  RndMeth=Zero
  Switch1 : Switch  Criteria=u2 ~= 0
  CC : Outport
  CC_en : Outport  Port=2
  SR : Outport  Port=3
  SR_en : Outport  Port=4
  wires:
  Data Type Conversion1/1 -> Map throttle into -1024..1023/1(in)
  Compare To Zero1/1 -> Logical Operator4/1
  Product/1 -> Detect Change/1, Build CAN CC message/1(CC)
  Map throttle into -1024..1023/1(out) -> Product/1
  Logical Operator4/1 -> Product/2
  Detect Change/1 -> CC_en/1, Logical Operator6/1
  Constant1/1 -> Switch1/1
  Constant2/1 -> Switch1/3
  RC Throttle/1 -> Compare To Zero1/1, Data Type Conversion1/1
  Detect to/from zero/2(changed) -> Logical Operator6/2
  Detect to/from zero/1(now zero) -> Switch1/2
  RC Rudder/1 -> Detect to/from zero/1(hightime)
  Switch1/1 -> SR/1
  Logical Operator6/1 -> SR_en/1
  Build CAN CC message/1(msg) -> CC/1

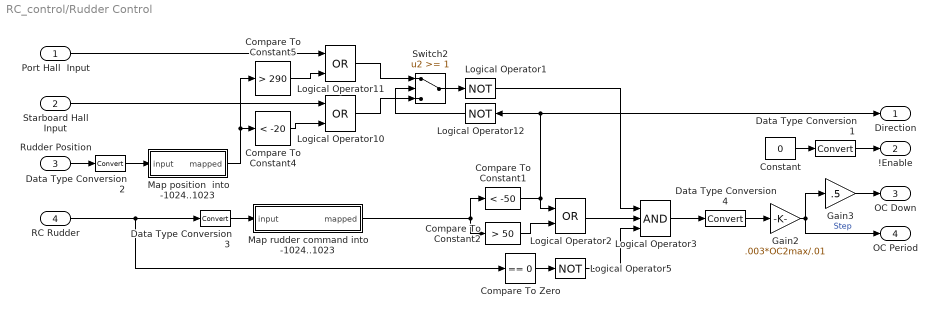
== system RC_control/Rudder Control ==
  Port Hall  Input : Inport
  Starboard Hall Input : Inport  Port=2
  Rudder Position : Inport  Port=3
  RC Rudder : Inport  Port=4
  Compare To Constant1 : simulink/Logic and Bit Operations/Compare To Constant  SystemSampleTime=-1  relop=<  const=-50  LogicOutDataTypeMode=boolean  ZeroCross=off
  Compare To Constant2 : simulink/Logic and Bit Operations/Compare To Constant  SystemSampleTime=-1  relop=>  const=50  LogicOutDataTypeMode=boolean  ZeroCross=off
  Compare To Constant4 : simulink/Logic and Bit Operations/Compare To Constant  SystemSampleTime=-1  relop=<  const=-20  LogicOutDataTypeMode=boolean  ZeroCross=off
  Compare To Constant5 : simulink/Logic and Bit Operations/Compare To Constant  SystemSampleTime=-1  relop=>  const=290  LogicOutDataTypeMode=boolean  ZeroCross=off
  Compare To Zero : simulink/Logic and Bit Operations/Compare To Zero  SystemSampleTime=-1  relop===  LogicOutDataTypeMode=boolean  ZeroCross=off
  Constant : Constant  Value=0
  Data Type Conversion1 : DataTypeConversion  OutDataTypeMode=boolean
  Data Type Conversion2 : DataTypeConversion  OutDataTypeMode=int16
  Data Type Conversion3 : DataTypeConversion  OutDataTypeMode=int16
  Data Type Conversion4 : DataTypeConversion
  Gain2 : Gain  Gain=.003*OC2max/.01
  Gain3 : Gain  Gain=.5
  Logical Operator1 : Logic  Operator=NOT  AllPortsSameDT=off  OutDataTypeMode=Boolean
  Logical Operator10 : Logic  Operator=OR  AllPortsSameDT=off  OutDataTypeMode=Boolean
  Logical Operator11 : Logic  Operator=OR  AllPortsSameDT=off  OutDataTypeMode=Boolean
  Logical Operator12 : Logic  Orientation=left  Operator=NOT  AllPortsSameDT=off  OutDataTypeMode=Boolean
  Logical Operator2 : Logic  Operator=OR  AllPortsSameDT=off  OutDataTypeMode=Boolean
  Logical Operator3 : Logic  Inputs=3  AllPortsSameDT=off  OutDataTypeMode=Specify via dialog
  Logical Operator5 : Logic  Operator=NOT  AllPortsSameDT=off  OutDataTypeMode=Boolean
  Map position  into -1024..1023 : Subsystem
  Map rudder command into -1024..1023 : Subsystem
  Switch2 : Switch  Threshold=1
  Direction : Outport
  !Enable : Outport  Port=2
  OC Down : Outport  Port=3
  OC Period : Outport  Port=4
  wires:
  Compare To Constant2/1 -> Logical Operator2/2
  Logical Operator2/1 -> Logical Operator3/2
  Logical Operator12/1 -> Switch2/2
  Switch2/1 -> Logical Operator1/1
  Logical Operator10/1 -> Switch2/3
  Logical Operator11/1 -> Switch2/1
  Logical Operator3/1 -> Data Type Conversion4/1
  Logical Operator1/1 -> Logical Operator3/1
  Data Type Conversion2/1 -> Map position  into -1024..1023/1(input)
  Map position  into -1024..1023/1(mapped) -> Compare To Constant5/1, Compare To Constant4/1
  Data Type Conversion3/1 -> Map rudder command into -1024..1023/1(input)
  Map rudder command into -1024..1023/1(mapped) -> Compare To Constant1/1, Compare To Constant2/1
  Compare To Constant5/1 -> Logical Operator11/2
  Compare To Constant4/1 -> Logical Operator10/2
  Logical Operator5/1 -> Logical Operator3/3
  Compare To Zero/1 -> Logical Operator5/1
  Data Type Conversion4/1 -> Gain2/1
  Compare To Constant1/1 -> Logical Operator12/1, Direction/1, Logical Operator2/1
  Gain2/1 -> Gain3/1, OC Period/1  "Step"
  RC Rudder/1 -> Data Type Conversion3/1, Compare To Zero/1
  Port Hall  Input/1 -> Logical Operator11/1
  Starboard Hall Input/1 -> Logical Operator10/1
  Rudder Position/1 -> Data Type Conversion2/1
  Gain3/1 -> OC Down/1
  Constant/1 -> Data Type Conversion1/1
  Data Type Conversion1/1 -> !Enable/1

== system RC_control/Drive Motor Speed Message/C-function Call ==
  parameters : Inport
  Enable : EnablePort
  ECAN1 Transmit [ecanFunctions.c] : dsPICdrivers/OTHERS/C Function Call  Tag=dsPIC_dsPIC_CFunctionCall  fctName='ecan1_transmit_matlab'  INPUT_SIZE=8  INPUT1=uint16  INPUT2=--  INPUT3=--  OUTPUT_SIZE=1  OUTPUT1=--  SampleTime=c_func_sample_time  InputType=[ 4 ]  OutputType=[ ]  FctDeclaration=extern void ecan1_transmit_matlab(uint16_T* u1);  FctCall=ecan1_transmit_matlab(*%u1);  OrderingInOutPopup=None
  Rate Transition : RateTransition
  wires:
  parameters/1 -> Rate Transition/1
  Rate Transition/1 -> ECAN1 Transmit [ecanFunctions.c]/1

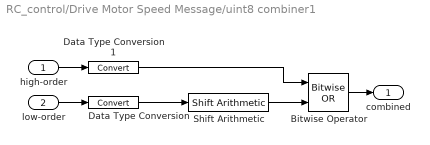
== system RC_control/Drive Motor Speed Message/uint8 combiner1 ==
  high-order : Inport
  low-order : Inport  Port=2
  Bitwise Operator : simulink/Logic and Bit Operations/Bitwise Operator  logicop=OR  UseBitMask=off  NumInputPorts=2  BitMask=bin2dec('11011001')  BitMaskRealWorld=Stored Integer
  Data Type Conversion : DataTypeConversion  OutDataTypeMode=uint16
  Data Type Conversion1 : DataTypeConversion  OutDataTypeMode=uint16
  Shift Arithmetic : simulink/Logic and Bit Operations/Shift Arithmetic  SystemSampleTime=-1  nBitShiftRight=-8  nBinPtShiftRight=0
  combined : Outport
  wires:
  Data Type Conversion1/1 -> Bitwise Operator/1
  Data Type Conversion/1 -> Shift Arithmetic/1
  Shift Arithmetic/1 -> Bitwise Operator/2
  high-order/1 -> Data Type Conversion1/1
  Bitwise Operator/1 -> combined/1
  low-order/1 -> Data Type Conversion/1

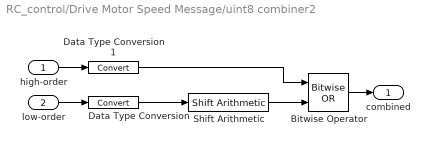
== system RC_control/Drive Motor Speed Message/uint8 combiner2 ==
  high-order : Inport
  low-order : Inport  Port=2
  Bitwise Operator : simulink/Logic and Bit Operations/Bitwise Operator  logicop=OR  UseBitMask=off  NumInputPorts=2  BitMask=bin2dec('11011001')  BitMaskRealWorld=Stored Integer
  Data Type Conversion : DataTypeConversion  OutDataTypeMode=uint16
  Data Type Conversion1 : DataTypeConversion  OutDataTypeMode=uint16
  Shift Arithmetic : simulink/Logic and Bit Operations/Shift Arithmetic  SystemSampleTime=-1  nBitShiftRight=-8  nBinPtShiftRight=0
  combined : Outport
  wires:
  low-order/1 -> Data Type Conversion/1
  Bitwise Operator/1 -> combined/1
  high-order/1 -> Data Type Conversion1/1
  Shift Arithmetic/1 -> Bitwise Operator/2
  Data Type Conversion/1 -> Shift Arithmetic/1
  Data Type Conversion1/1 -> Bitwise Operator/1

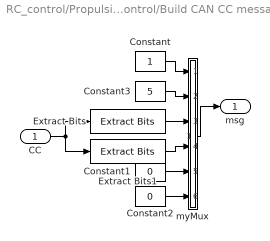
== system RC_control/Propulsion Control/Build CAN CC message ==
  CC : Inport
  Constant : Constant
  Constant1 : Constant  Value=0
  Constant2 : Constant  Value=0
  Constant3 : Constant  Value=5
  Extract Bits : simulink/Logic and Bit Operations/Extract Bits  SystemSampleTime=-1  bitsToExtract=Upper half  numBits=8  bitIdxRange=[0 7]  outScalingMode=Preserve fixed-point scaling
  Extract Bits1 : simulink/Logic and Bit Operations/Extract Bits  SystemSampleTime=-1  bitsToExtract=Lower half  numBits=8  bitIdxRange=[0 7]  outScalingMode=Preserve fixed-point scaling
  myMux : Stateflow chart
  msg : Outport
  wires:
  Constant/1 -> myMux/1(u1)
  Constant3/1 -> myMux/2(u2)
  CC/1 -> Extract Bits1/1, Extract Bits/1
  Extract Bits/1 -> myMux/3(u3)
  Extract Bits1/1 -> myMux/4(u4)
  myMux/1(y) -> msg/1
  Constant1/1 -> myMux/5(u5)
  Constant2/1 -> myMux/6(u6)
